simulink model "SF027A_EotProtnFwl"  (R2013b)
settings: Solver=FixedStepDiscrete  SolverMode=SingleTasking  StartTime=0.0  StopTime=1  FixedStep=0.002  RelTol=1e-3
undefined symbols (not defined in the file): ACTVREGN_CNT_U08, ARCHGLBPRM_FLOATZEROTHD_ULS_F32, EOTACTVCMDFWLREACHED_CNT_U08, EOTDMPGFWLREACHED_CNT_U08, EotProtnFwlInactvLim, EotProtnHwAgMin, EotProtnHwDegDampgX, EotProtnRackTrvlLimrRng, EotProtnSoftEndStopAuthyThd, FWLDISAD_CNT_U08, INACTVREGN_CNT_U08, MfgEnaSt1, NtcNr1, NtcSts1, sigbuilder_block
libraries: simulink x8, NxtrLim x6, FixdToFloat x5, LnrIntrpn x2, BilnrIntrpnCmnX x2, FloatToFixd x2, NxtrAbslt x1
(part 1 of 2)
Description:
  | This function sums and bounds motor torque commands from system functions whose primary input is handwheel torque.  After summation, output is limited when the signal's low-frequency content
  | exceeds calibrated boundaries.  If undesired behavior persists,  the signal-limiting strategy is replaced with implementation of a simple default assist table lookup.  Switching limiter to default table
  | occurs via Pstep/Nstep counter.  The function also outputs a scale factor for the application of additional damping.     This Function requires SF-00 Common Calibrations.
settings Model: Creator=lzz0tm  LastModifiedBy=fzx0rm
settings Model: ModifiedHistory=|
  | 001
  | Initial release
  | K. Derry
  | 18-Apr-2012
  | ICR 3358
  | 
  | 002
  | 1.  Added three limiters, applied to incoming Hysteresis_Comp, HighFreqAssist, and BaseAssistCmd.
  | 2. Created three new calibrations for input limiters.
  | 3. Increased range of boundary cals from +/- 8.8 to +/-16.
  | K. Derry
  | 31-May-2012
  | ICR 3467
  | 
  | 003
  | Extensive logic changes in model.
  | Four additional display variables.
  | K. Derry
  | 7-Jun-2012
  | ICR 3479
  | 
  | 004
  | Added logic to change AssistActiveRaw to zero when PstepNstep counter reaches saturation.
  | Changed PN Counter IF..THEN logic from “>=” to “>”.
  | K. Derry
  | 20-Jun-2012
  | ICR-3541
  | 
  | 005
  | 1. Logic now transitions output from a boundary-limited value to a default assist table lookup.
  | 2. Added new display variables.
  | 3. Increase range of boundary cals from +/-8.8 to +/-16.
  | K. Derry
  | 23-Jul-2012
  | ICR-3602
  | 
  | 006
  | Changed range & resolution of default assist cals to match Assist tables.
  | K. Derry
  | 31-Jul-2012
  | anom 3594
  | 
  | 007
  | Reduce table size and cal only quadrants 1 and 2, calculating 3 and 4.
  | Add NTC outputs to FDD to match existing code.
  | Modify model layout to better match existing code.
  | Use common vehicle speed table.
  | Eliminate Word doc.
  | K. Derry
  | 23-Jan-2013
  | ICR-3927
  | 
  | 008
  | Add inputs and logic to defeat firewall when SF-01 is using linear gain table.
  | Replace 1x12 'Cmn_t_VehSpd_Kph' with 1x8 'AsstFW_t_VehSpd_kph'.
  | Resize boundary tables to 8 vehicle speeds.
  | S. Millsap
  | K. Derry
  | 30-Apr-2013
  | ICR-4102
  | 
  | 009
  | Change rates & states execution requirement from Optional to Do Not Execute for Warm Init
  | and Disable
  | S. Millsap
  | 12-Nov-14
  | ICR-4722
settings SolverCC: AutoInsertRateTranBlk=on  InsertRTBMode=Always
settings DataIOCC: LimitDataPoints=off  SaveFormat=Structure  ReturnWorkspaceOutputs=on
settings OptimizationCC: BlockReduction=off  InlineParams=on  ZeroExternalMemoryAtStartup=off  ZeroInternalMemoryAtStartup=off  OptimizeModelRefInitCode=on  LifeSpan=1
settings DebuggingCC: SignalInfNanChecking=error  SignalRangeChecking=warning  UnderspecifiedInitializationDetection=Simplified  SolverPrmCheckMsg=error  InheritedTsInSrcMsg=error  DiscreteInheritContinuousMsg=error  SingleTaskRateTransMsg=error  TasksWithSamePriorityMsg=error  SigSpecEnsureSampleTimeMsg=error  CheckMatrixSingularityMsg=error  ParameterUnderflowMsg=error  ParameterPrecisionLossMsg=error  ParameterTunabilityLossMsg=error  FixptConstUnderflowMsg=warning  FixptConstOverflowMsg=warning  VectorMatrixConversionMsg=error  SignalLabelMismatchMsg=error  UnconnectedInputMsg=error  UnconnectedOutputMsg=error  UnconnectedLineMsg=error  SFcnCompatibilityMsg=error  UniqueDataStoreMsg=warning  BusObjectLabelMismatch=error  RootOutportRequireBusObject=error  AssertControl=DisableAll  ModelReferenceIOMsg=error  ModelReferenceVersionMismatchMessage=warning  ModelReferenceIOMismatchMessage=error  ModelReferenceCSMismatchMessage=warning  ModelReferenceDataLoggingMessage=error  StateNameClashWarn=warning  StrictBusMsg=ErrorOnBusTreatedAsVector  NonBusSignalsTreatedAsBus=error  SFUnexpectedBacktrackingDiag=error  SFInvalidInputDataAccessInChartInitDiag=error  SFNoUnconditionalDefaultTransitionDiag=error  SFTransitionOutsideNaturalParentDiag=error  SFUnconditionalTransitionShadowingDiag=error  SFUndirectedBroadcastEventsDiag=error
settings ModelReferenceCC: ModelReferenceNumInstancesAllowed=Single
settings RTWCC: SystemTargetFile=autosar.tlc  GenCodeOnly=on  TemplateMakefile=ert_default_tmf  Description=AUTOSAR  GenerateReport=on  ProcessScript=autosar_make_rtw_hook  LaunchReport=on
settings CodeAppCC: GenerateComments=off  IgnoreCustomStorageClasses=off  CustomSymbolStrType=$N$R$M  CustomSymbolStrBlkIO=$N$M  SimulinkBlockComments=off
settings STFCustomTargetCC: ParMdlRefBuildCompliant=on  CompOptLevelCompliant=on  IncludeMdlTerminateFcn=off  CombineOutputUpdateFcns=on  SuppressErrorStatus=on  ERTFirstTimeCompliant=on  ERTCustomFileBanners=on  SupportNonFinite=off  SupportComplex=off  SupportContinuousTime=off  SupportNonInlinedSFcns=off  MATLABClassNameForMDSCustomization=Simulink.SoftwareTarget.ERTCustomization  AutosarCompliant=on  GRTInterface=off  SystemTargetFile=autosar.tlc
settings ERTTargetCC: CodeReplacementLibrary=ANSI_C  ConcurrentExecutionCompliant=off  IncludeMdlTerminateFcn=off  SuppressErrorStatus=on  SupportNonFinite=off  SupportComplex=off  ModelStepFunctionPrototypeControlCompliant=off  CPPClassGenCompliant=off  AutosarCompliant=on  InlinedParameterPlacement=NonHierarchical  ERTCustomFileTemplate=example_file_process.tlc  EnableUserReplacementTypes=on

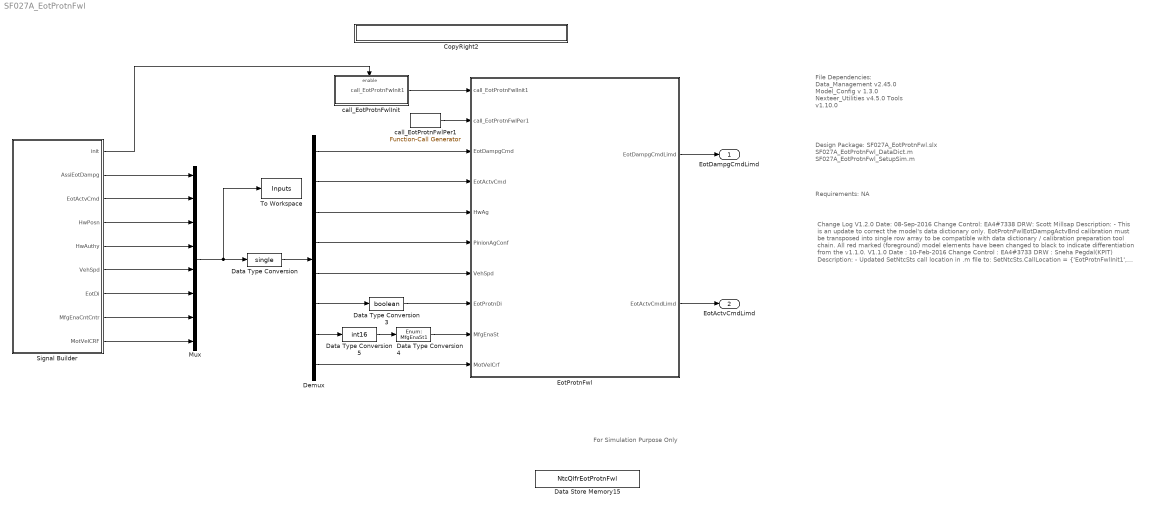
== system SF027A_EotProtnFwl ==
  note: File Dependencies:
      |
      | Data_Management v2.45.0
      | Model_Config v 1.3.0
      | Nexteer_Utilities v4.5.0
      | Tools v1.10.0
  note: Design Package:
      | SF027A_EotProtnFwl.slx
      | SF027A_EotProtnFwl_DataDict.m
      | SF027A_EotProtnFwl_SetupSim.m
  note: Change Log
      | V1.2.0
      | Date: 08-Sep-2016
      | Change Control: EA4#7338
      | DRW: Scott Millsap
      | Description:
      | - This is an update to correct the model's data dictionary only. EotProtnFwlEotDampgActvBnd
      | calibration must be transposed into single row array to be compatible with data dictionary /
      | calibration preparation tool chain.   All red marked (foreground) model elements have been changed to
      | black to indicate differentiation from the v1.1.0.
      | V1.1.0
      | Date : 10-Feb-2016
      | Change Control : EA4#3733
      | DRW : Sneha Pegdal(KPIT)
      | Description:
      | - Updated SetNtcSts call location in .m file to:
      | SetNtcSts.CallLocation = {'EotProtnFwlInit1', 'EotProtnFwlPer1'};
      | - Created an output "EotDampgFwlReached' (assigned with value 'false')
      |  from "Defeat Firewall" (If) subsystemand linked it to merge block.
      | - Renamed output "EotDampgFwlOverBnd" of "EotDmpActiveRegion"
      |   (ElseIf) subsystem to "EotDampgFwlReached'.
      | - Created an output "EotActvCmdFwlReached' (assigned with value 'false')
      |   from "Defeat Firewall1" (If) subsystem and linked it to merge block.
      | - In "Set_Faults" subsystem, removed conversion from bool to unit8. Modified logic of setting "NtcStInfo".
      |
      | Ver: 1.0.0
      | Author : KeyurKumar Gondaliya(KPIT)
      | Date : 25-Jan-2016
      | ICR- EA4#3059
      | - EA4 Initial Version from EA3 v4.0.X
  note: Requirements: NA
  note: For Simulation Purpose Only
  CopyRight2 : Subsystem  Description=|  mask(Copyright Information){none=on}
      | Copyright info block.                                               
      |                                                                     
      | Place copyright information at the top of every subsystem in design.
      mask prompts: none "No parameters"
      mask help: Place copyright information at the top of every subsystem in design.
      mask Display:
      | NxtrConf = 'Nexteer Confidential';
      | 
      | sys = bdroot; %handle for the current model ("system")
      | first = get_param(sys,'Created');
      | first = first(end-3:end);  %year is last four digits
      | 
      | last = get_param(sys,'LastModifiedDate');
      | if isempty(last)
      |     last = datestr(now,'yyyy');
      | else
      |     last = last(end-3:end);
      | end
      | 
      | if strcmp(first,last)
      |     fprintf('%s -- Copyright %s Nexteer',NxtrConf,first)
      | else
      |     fprintf('%s -- %s%s- %s Nexteer',NxtrConf,char(169),first,last)
      | end
  Data Store Memory15 : DataStoreMemory  DataStoreName=NtcQlfrEotProtnFwl  InitialValue=SigQlfr1.SIGQLFR_PASSD  OutDataTypeStr=Enum: SigQlfr1
  Data Type Conversion : DataTypeConversion  OutDataTypeStr=single
  Data Type Conversion3 : DataTypeConversion  OutDataTypeStr=boolean
  Data Type Conversion4 : DataTypeConversion  OutDataTypeStr=Enum: MfgEnaSt1
  Data Type Conversion5 : DataTypeConversion  OutDataTypeStr=int16
  Demux : Demux  Outputs=8
  EotProtnFwl : Subsystem
  Mux : Mux  Inputs=8
  Signal Builder : Subsystem  Tag=STV Subsys  LoadFcn=sigbuilder_block('load');  StartFcn=sigbuilder_block('start');  StopFcn=sigbuilder_block('stop');  ClipboardFcn=sigbuilder_block('clipboard');  mask(Sigbuilder block){}
      mask help: Simulink:masks:SigbuilderBlock_MD
      mask init:
      | if ~strcmp(get_param(bdroot(gcbh),'SimulationStatus'),'stopped') tuvar = sigbuilder_block('maskInit'); end
      settings: CopyFcn=sigbuilder_block('copy');  DeleteFcn=sigbuilder_block('delete');  ModelCloseFcn=sigbuilder_block('modelClose');  PreSaveFcn=sigbuilder_block('preSave');  PauseFcn=sigbuilder_block('pause');  ContinueFcn=sigbuilder_block('continue');  NameChangeFcn=sigbuilder_block('namechange');  OpenFcn=sigbuilder_block('open',[55.5 0 1204.5 730.5 ]);  CloseFcn=sigbuilder_block('close');
      mask Display: plot(0, 0, 100, 100,[2, 2, 32, 32, 2], [68, 8, 8, 68, 68],[32, 2], [38, 38], [32, 19, 2],[53, 60, 44], [32, 17, 17, 2],[16, 16, 31, 31]);txt = getActiveGroup(gcbh);text(2, 100, txt,'verticalAlignment', 'top');
  To Workspace : ToWorkspace  VariableName=Inputs  SampleTime=-1
  call_EotProtnFwlInit : Subsystem  TreatAsAtomicUnit=on
  call_EotProtnFwlPer1 : simulink/Ports & Subsystems/Function-Call Generator  RequirementInfo={} %GIDa_97dce53d_9879_4c16_9f7c_2c76ae6021b7  sample_time=0.002  numberOfIterations=1
  EotDampgCmdLimd : Outport
  EotActvCmdLimd : Outport  Port=2
  wires:
  call_EotProtnFwlPer1/1 -> EotProtnFwl/2(call_EotProtnFwlPer1)
  EotProtnFwl/1(EotDampgCmdLimd) -> EotDampgCmdLimd/1
  EotProtnFwl/2(EotActvCmdLimd) -> EotActvCmdLimd/1
  call_EotProtnFwlInit/1(call_EotProtnFwInit1) -> EotProtnFwl/1(call_EotProtnFwlInit1)
  Mux/1 -> To Workspace/1, Data Type Conversion/1
  Signal Builder/1(init) -> call_EotProtnFwlInit/Enable
  Signal Builder/5(HwAuthy) -> Mux/4
  Signal Builder/6(VehSpd) -> Mux/5
  Signal Builder/4(HwPosn) -> Mux/3
  Signal Builder/7(EotDi) -> Mux/6
  Signal Builder/3(EotActvCmd) -> Mux/2
  Signal Builder/8(MfgEnaCntCntr) -> Mux/7
  Signal Builder/2(AssiEotDampg) -> Mux/1
  Signal Builder/9(MotVelCRF) -> Mux/8
  Demux/1 -> EotProtnFwl/3(EotDampgCmd)
  Demux/2 -> EotProtnFwl/4(EotActvCmd)
  Demux/3 -> EotProtnFwl/5(HwAg)
  Demux/4 -> EotProtnFwl/6(PinionAgConf)
  Demux/5 -> EotProtnFwl/7(VehSpd)
  Demux/6 -> Data Type Conversion3/1
  Demux/7 -> Data Type Conversion5/1
  Demux/8 -> EotProtnFwl/10(MotVelCrf)
  Data Type Conversion/1 -> Demux/1
  Data Type Conversion3/1 -> EotProtnFwl/8(EotProtnDi)
  Data Type Conversion4/1 -> EotProtnFwl/9(MfgEnaSt)
  Data Type Conversion5/1 -> Data Type Conversion4/1

== system SF027A_EotProtnFwl/CopyRight2 ==

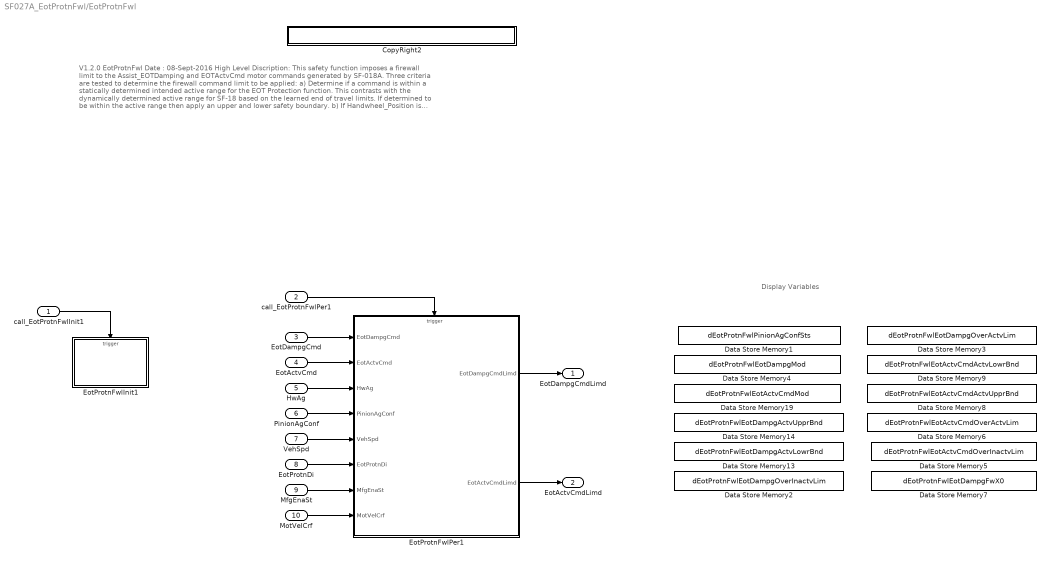
== system SF027A_EotProtnFwl/EotProtnFwl ==
  note: Display Variables
  note: V1.2.0    EotProtnFwl                                                                                                                                  Date : 08-Sept-2016
      |
      | High Level Discription:
      |
      | This safety function imposes a firewall limit to the Assist_EOTDamping and EOTActvCmd motor commands generated by SF-018A.
      |
      |  Three criteria are tested to determine the firewall command limit to be applied:
      | a) Determine if a command is within a statically determined intended active range for the EOT Protection function.  This contrasts with the
      | dynamically determined active range for SF-18 based on the learned end of travel limits. If determined to be within the active range then apply
      | an upper and lower safety boundary.
      | b) If Handwheel_Position is inboard of the active region (e.g. between +/- X0), then apply simple saturation limit.
      | c) If Handwheel_Authority is below a calibration threshold value, then apply simple saturation limit.
  call_EotProtnFwlInit1 : Inport
  call_EotProtnFwlPer1 : Inport  Port=2
  EotDampgCmd : Inport  Port=3
  EotActvCmd : Inport  Port=4
  HwAg : Inport  Port=5
  PinionAgConf : Inport  Port=6
  VehSpd : Inport  Port=7
  EotProtnDi : Inport  Port=8
  MfgEnaSt : Inport  Port=9
  MotVelCrf : Inport  Port=10
  CopyRight2 : Subsystem  Description=|  mask(Copyright Information){none=on}
      | Copyright info block.                                               
      |                                                                     
      | Place copyright information at the top of every subsystem in design.
      mask prompts: none "No parameters"
      mask help: Place copyright information at the top of every subsystem in design.
      mask Display:
      | NxtrConf = 'Nexteer Confidential';
      | 
      | sys = bdroot; %handle for the current model ("system")
      | first = get_param(sys,'Created');
      | first = first(end-3:end);  %year is last four digits
      | 
      | last = get_param(sys,'LastModifiedDate');
      | if isempty(last)
      |     last = datestr(now,'yyyy');
      | else
      |     last = last(end-3:end);
      | end
      | 
      | if strcmp(first,last)
      |     fprintf('%s -- Copyright %s Nexteer',NxtrConf,first)
      | else
      |     fprintf('%s -- %s%s- %s Nexteer',NxtrConf,char(169),first,last)
      | end
  Data Store Memory1 : DataStoreMemory  DataStoreName=dEotProtnFwlPinionAgConfSts  OutDataTypeStr=boolean  StateMustResolveToSignalObject=on
  Data Store Memory13 : DataStoreMemory  DataStoreName=dEotProtnFwlEotDampgActvLowrBnd  OutDataTypeStr=single  StateMustResolveToSignalObject=on
  Data Store Memory14 : DataStoreMemory  DataStoreName=dEotProtnFwlEotDampgActvUpprBnd  OutDataTypeStr=single  StateMustResolveToSignalObject=on
  Data Store Memory19 : DataStoreMemory  DataStoreName=dEotProtnFwlEotActvCmdMod  OutDataTypeStr=uint8  StateMustResolveToSignalObject=on
  Data Store Memory2 : DataStoreMemory  DataStoreName=dEotProtnFwlEotDampgOverInactvLim  OutDataTypeStr=boolean  StateMustResolveToSignalObject=on
  Data Store Memory3 : DataStoreMemory  DataStoreName=dEotProtnFwlEotDampgOverActvLim  OutDataTypeStr=boolean  StateMustResolveToSignalObject=on
  Data Store Memory4 : DataStoreMemory  DataStoreName=dEotProtnFwlEotDampgMod  OutDataTypeStr=uint8  StateMustResolveToSignalObject=on
  Data Store Memory5 : DataStoreMemory  DataStoreName=dEotProtnFwlEotActvCmdOverInactvLim  OutDataTypeStr=boolean  StateMustResolveToSignalObject=on
  Data Store Memory6 : DataStoreMemory  DataStoreName=dEotProtnFwlEotActvCmdOverActvLim  OutDataTypeStr=boolean  StateMustResolveToSignalObject=on
  Data Store Memory7 : DataStoreMemory  DataStoreName=dEotProtnFwlEotDampgFwX0  StateMustResolveToSignalObject=on
  Data Store Memory8 : DataStoreMemory  DataStoreName=dEotProtnFwlEotActvCmdActvUpprBnd  OutDataTypeStr=single  StateMustResolveToSignalObject=on
  Data Store Memory9 : DataStoreMemory  DataStoreName=dEotProtnFwlEotActvCmdActvLowrBnd  OutDataTypeStr=single  StateMustResolveToSignalObject=on
  EotProtnFwlInit1 : Subsystem  TreatAsAtomicUnit=on
  EotProtnFwlPer1 : Subsystem
  EotDampgCmdLimd : Outport
  EotActvCmdLimd : Outport  Port=2
  wires:
  call_EotProtnFwlInit1/1 -> EotProtnFwlInit1/Trigger
  call_EotProtnFwlPer1/1 -> EotProtnFwlPer1/Trigger
  EotProtnFwlPer1/1(EotDampgCmdLimd) -> EotDampgCmdLimd/1
  EotProtnFwlPer1/2(EotActvCmdLimd) -> EotActvCmdLimd/1
  EotDampgCmd/1 -> EotProtnFwlPer1/1(EotDampgCmd)
  EotActvCmd/1 -> EotProtnFwlPer1/2(EotActvCmd)
  HwAg/1 -> EotProtnFwlPer1/3(HwAg)
  PinionAgConf/1 -> EotProtnFwlPer1/4(PinionAgConf)
  VehSpd/1 -> EotProtnFwlPer1/5(VehSpd)
  EotProtnDi/1 -> EotProtnFwlPer1/6(EotProtnDi)
  MfgEnaSt/1 -> EotProtnFwlPer1/7(MfgEnaSt)
  MotVelCrf/1 -> EotProtnFwlPer1/8(MotVelCrf)

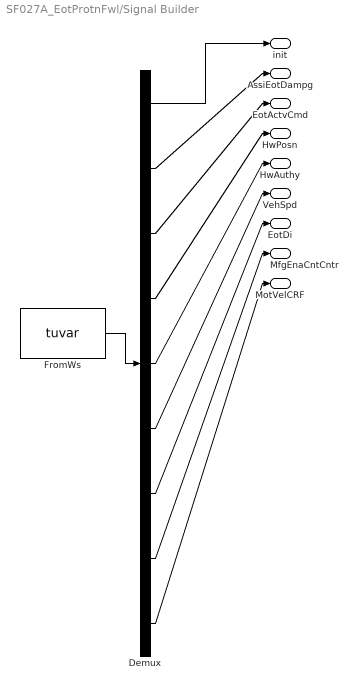
== system SF027A_EotProtnFwl/Signal Builder ==
  Demux : Demux  Tag=STV Demux  Outputs=9
  FromWs : FromWorkspace  Tag=STV FromWs  VariableName=tuvar  SampleTime=0
      SigBuilderData=|
      | common.afterFinalStr = 'Extrapolate'
      | common.sampleTime = 0
      | dataSet.timeRange = [0 5]
      | dataSet.name = 'SF027A_EotProtnFw'
      | sbobj.Name = 'Signal Builder'
      | sbobj.Groups.Name = 'SF027A_EotProtnFw'
      | sbobj.Groups.Signals(1).Name = 'init'
      | sbobj.Groups.Signals(1).XData = [0 0.002 0.004 0.006 0.008 0.01 0.012 0.014 0.016 0.018 0.02 0.022 ... (2501 elements, 1x2501)]
      | sbobj.Groups.Signals(1).YData = [1 0 0 0 0 0 0 0 0 0 0 0 ... (2501 elements, 1x2501)]
      | sbobj.Groups.Signals(2).Name = 'AssiEotDampg'
      | sbobj.Groups.Signals(2).XData = [0 0.002 0.004 0.006 0.008 0.01 0.012 0.014 0.016 0.018 0.02 0.022 ... (2501 elements, 1x2501)]
      | sbobj.Groups.Signals(2).YData = [0 0.0175999882667 0.0351999061334 0.0527996832006 0.0703992490691 0.0879985333407 0.105597465618 0.123195975506 0.14079399261 0.158391446539 0.175988266901 0.193584383311 ... (2501 elements, 1x2501)]
      | sbobj.Groups.Signals(3).Name = 'EotActvCmd'
      | sbobj.Groups.Signals(3).XData = [0 0.002 0.004 0.006 0.008 0.01 0.012 0.014 0.016 0.018 0.02 0.022 ... (2501 elements, 1x2501)]
      | sbobj.Groups.Signals(3).YData = [0 0.0175999882667 0.0351999061334 0.0527996832006 0.0703992490691 0.0879985333407 0.105597465618 0.123195975506 0.14079399261 0.158391446539 0.175988266901 0.193584383311 ... (2501 elements, 1x2501)]
      | sbobj.Groups.Signals(4).Name = 'HwPosn'
      | sbobj.Groups.Signals(4).XData = [0 0.002 0.004 0.006 0.008 0.01 0.012 0.014 0.016 0.018 0.02 0.022 ... (2501 elements, 1x2501)]
      | sbobj.Groups.Signals(4).YData = [0 2.87999808 5.75998464001 8.63994816009 11.5198771204 14.3997600012 17.279585283 20.1593414465 23.0390169726 25.9186003427 28.7980800384 31.6774445418 ... (2501 elements, 1x2501)]
      | sbobj.Groups.Signals(5).Name = 'HwAuthy'
      | sbobj.Groups.Signals(5).XData = [0 0.002 0.004 0.006 0.008 0.01 0.012 0.014 0.016 0.018 0.02 0.022 ... (2501 elements, 1x2501)]
      | sbobj.Groups.Signals(5).YData = [0 1 0 1 0 1 0 1 0 1 0 1 ... (2501 elements, 1x2501)]
      | sbobj.Groups.Signals(6).Name = 'VehSpd'
      | sbobj.Groups.Signals(6).XData = [0 0.002 0.004 0.006 0.008 0.01 0.012 0.014 0.016 0.018 0.02 0.022 ... (2501 elements, 1x2501)]
      | sbobj.Groups.Signals(6).YData = [1.02199931867 2.04399454934 3.06598160403 4.08795639481 5.10991483376 6.13185283306 7.15376630496 8.1756511618 9.19750331605 10.2193186803 11.2410931673 12.2628226899 ... (2501 elements, 1x2501)]
      | sbobj.Groups.Signals(7).Name = 'EotDi'
      | sbobj.Groups.Signals(7).XData = [0 0.002 0.004 0.006 0.008 0.01 0.012 0.014 0.016 0.018 0.02 0.022 ... (2501 elements, 1x2501)]
      | sbobj.Groups.Signals(7).YData = [0 1 0 1 0 1 0 1 0 1 0 1 ... (2501 elements, 1x2501)]
      | sbobj.Groups.Signals(8).Name = 'MfgEnaCntCntr'
      | sbobj.Groups.Signals(8).XData = [0 2 2 3 3 5]
      | sbobj.Groups.Signals(8).YData = [0 0 1 1 0 0]
      | sbobj.Groups.Signals(9).Name = 'MotVelCRF'
      | sbobj.Groups.Signals(9).XData = [0 0.002 0.004 0.006 0.008 0.01 0.012 0.014 0.016 0.018 0.02 0.022 ... (2501 elements, 1x2501)]
      | sbobj.Groups.Signals(9).YData = [2.23599850933 4.47198807468 6.70795975207 8.94390459764 11.1798136676 13.4156780183 15.6514887063 17.8872367884 20.1229133216 22.3585093631 24.5940159707 26.8294242022 ... (2501 elements, 1x2501)]
      | sbobj.Groups.TimeRange = [0 5]
  init : Outport
  AssiEotDampg : Outport  Tag=STV Outport  Port=2
  EotActvCmd : Outport  Tag=STV Outport  Port=3
  HwPosn : Outport  Tag=STV Outport  Port=4
  HwAuthy : Outport  Tag=STV Outport  Port=5
  VehSpd : Outport  Tag=STV Outport  Port=6
  EotDi : Outport  Tag=STV Outport  Port=7
  MfgEnaCntCntr : Outport  Tag=STV Outport  Port=8
  MotVelCRF : Outport  Tag=STV Outport  Port=9
  wires:
  Demux/1 -> init/1
  FromWs/1 -> Demux/1
  Demux/2 -> AssiEotDampg/1
  Demux/3 -> EotActvCmd/1
  Demux/4 -> HwPosn/1
  Demux/5 -> HwAuthy/1
  Demux/6 -> VehSpd/1
  Demux/7 -> EotDi/1
  Demux/8 -> MfgEnaCntCntr/1
  Demux/9 -> MotVelCRF/1

== system SF027A_EotProtnFwl/call_EotProtnFwlInit ==
  Enable : EnablePort
  CopyRight2 : Subsystem  Description=|  mask(Copyright Information){none=on}
      | Copyright info block.                                               
      |                                                                     
      | Place copyright information at the top of every subsystem in design.
      mask prompts: none "No parameters"
      mask help: Place copyright information at the top of every subsystem in design.
      mask Display:
      | NxtrConf = 'Nexteer Confidential';
      | 
      | sys = bdroot; %handle for the current model ("system")
      | first = get_param(sys,'Created');
      | first = first(end-3:end);  %year is last four digits
      | 
      | last = get_param(sys,'LastModifiedDate');
      | if isempty(last)
      |     last = datestr(now,'yyyy');
      | else
      |     last = last(end-3:end);
      | end
      | 
      | if strcmp(first,last)
      |     fprintf('%s -- Copyright %s Nexteer',NxtrConf,first)
      | else
      |     fprintf('%s -- %s%s- %s Nexteer',NxtrConf,char(169),first,last)
      | end
  call_EotProtnFwInit : simulink/Ports & Subsystems/Function-Call Generator  sample_time=0  numberOfIterations=1
  call_EotProtnFwInit1 : Outport
  wires:
  call_EotProtnFwInit/1 -> call_EotProtnFwInit1/1

== system SF027A_EotProtnFwl/EotProtnFwl/CopyRight2 ==

== system SF027A_EotProtnFwl/EotProtnFwl/EotProtnFwlInit1 ==
  note: NEXTEER TROUBLE CODES
      |
      | Number                TYPE                   Name
      | NTCNR_0X0C6      F3      NTCNumber.NTC_EotProtnFwlFlt
  function : TriggerPort  TriggerType=function-call
  Constant7 : Constant  RequirementInfo={} %GIDa_126a797a_30b9_4b52_8911_b7affaa2f3a8  Value=0  OutDataTypeStr=uint8
  CopyRight2 : Subsystem  Description=|  mask(Copyright Information){none=on}
      | Copyright info block.                                               
      |                                                                     
      | Place copyright information at the top of every subsystem in design.
      mask prompts: none "No parameters"
      mask help: Place copyright information at the top of every subsystem in design.
      mask Display:
      | NxtrConf = 'Nexteer Confidential';
      | 
      | sys = bdroot; %handle for the current model ("system")
      | first = get_param(sys,'Created');
      | first = first(end-3:end);  %year is last four digits
      | 
      | last = get_param(sys,'LastModifiedDate');
      | if isempty(last)
      |     last = datestr(now,'yyyy');
      | else
      |     last = last(end-3:end);
      | end
      | 
      | if strcmp(first,last)
      |     fprintf('%s -- Copyright %s Nexteer',NxtrConf,first)
      | else
      |     fprintf('%s -- %s%s- %s Nexteer',NxtrConf,char(169),first,last)
      | end
  Enumerated Constant4 : simulink/Sources/Enumerated Constant  RequirementInfo={} %GIDa_605febc4_2a20_461f_8109_182131f61dc1  OutDataTypeStr=Enum: NtcSts1  Value=NtcSts1.NTCSTS_PASSD  SampleTime=inf
  EotProtnFwlFlt : simulink/Sources/Enumerated Constant  RequirementInfo={} %GIDa_6290572b_f437_4fd8_9e79_bb4e9500ca68  OutDataTypeStr=Enum: NtcNr1  Value=NtcNr1.NTCNR_0X0C6  SampleTime=inf
  Ground : Ground
  SetNtcSts : Subsystem  mask(SetNTC){}
      mask help: SetNTC library block
  wires:
  EotProtnFwlFlt/1 -> SetNtcSts/1(NtcNr)
  Constant7/1 -> SetNtcSts/2(NtcStInfo)
  Enumerated Constant4/1 -> SetNtcSts/3(NtcSts)
  Ground/1 -> SetNtcSts/4(DebStep)

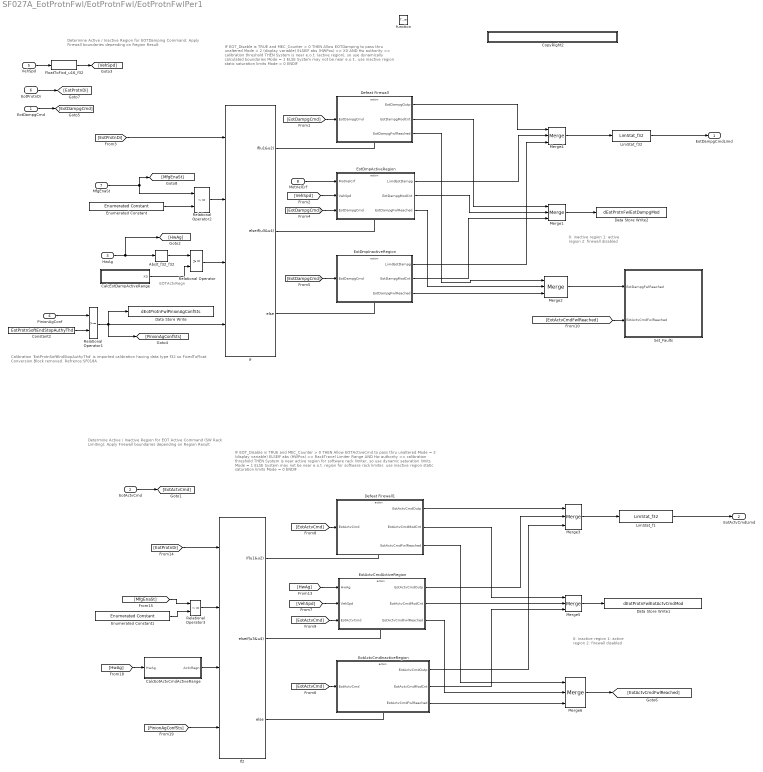
== system SF027A_EotProtnFwl/EotProtnFwl/EotProtnFwlPer1 ==
  note: Calibration 'EotProtnSoftEndStopAuthyThd' is imported calibration having data type f32 so FixedToFloat
      | Conversion Block removed.
      |
      | Refrence:SF018A
  note: EOTActvRegn
  note: 0: inactive region
      | 1: active region
      | 2: firewall disabled
  note: IF EOT_Disable is TRUE and MEC_Counter > 0 THEN
      |      Allow EOTDamping  to pass thru unaltered
      |      Mode = 2 (display variable)
      | ELSEIF abs (HWPos) >= X0   AND   Hw authority >= calibration threshold THEN
      |      System is near e.o.t. (active region), so use dynamically calculated boundaries
      |      Mode = 1
      | ELSE
      |      System may not be near e.o.t., use inactive region static saturation limits
      |      Mode = 0
      | ENDIF
  note: IF EOT_Disable is TRUE and MEC_Counter > 0 THEN
      |      Allow EOTActiveCmd  to pass thru unaltered
      |      Mode = 2 (display variable)
      | ELSEIF abs (HWPos) >= RackTravel Limiter Range   AND  Hw authority >= calibration threshold THEN
      |      System is near active region for software rack limiter, so use dynamic saturation limits
      |      Mode = 1
      | ELSE
      |      System may not be near e.o.t. region for software rack limiter, use inactive region static saturation limits
      |      Mode = 0
      | ENDIF
  note: Determine Active / Inactive Region for
      | EOTDamping Command; Apply Firewall boundaries
      | depending on Region Result
  note: Determine Active / Inactive Region for
      | EOT Active Command (SW Rack Limiting);
      | Apply Firewall boundaries depending on Region Result
  note: 0: inactive region
      | 1: active region
      | 2: firewall disabled
  EotDampgCmd : Inport
  EotActvCmd : Inport  Port=2
  HwAg : Inport  Port=3
  PinionAgConf : Inport  Port=4
  VehSpd : Inport  Port=5
  EotProtnDi : Inport  Port=6
  MfgEnaSt : Inport  Port=7
  MotVelCrf : Inport  Port=8
  function : TriggerPort  TriggerType=function-call
  Abslt_f32_f32 : NxtrAbslt/Abslt_f32_f32  SFunctionSpec=single y1 = Abslt_f32_f32(single u1)
      settings: AttributesFormatString=%<Name>
  CalcEotActvCmdActiveRange : Subsystem
  CalcEotDampActiveRange : Subsystem
  Constant2 : Constant  Value=EotProtnSoftEndStopAuthyThd
  CopyRight2 : Subsystem  Description=|  mask(Copyright Information){none=on}
      | Copyright info block.                                               
      |                                                                     
      | Place copyright information at the top of every subsystem in design.
      mask prompts: none "No parameters"
      mask help: Place copyright information at the top of every subsystem in design.
      mask Display:
      | NxtrConf = 'Nexteer Confidential';
      | 
      | sys = bdroot; %handle for the current model ("system")
      | first = get_param(sys,'Created');
      | first = first(end-3:end);  %year is last four digits
      | 
      | last = get_param(sys,'LastModifiedDate');
      | if isempty(last)
      |     last = datestr(now,'yyyy');
      | else
      |     last = last(end-3:end);
      | end
      | 
      | if strcmp(first,last)
      |     fprintf('%s -- Copyright %s Nexteer',NxtrConf,first)
      | else
      |     fprintf('%s -- %s%s- %s Nexteer',NxtrConf,char(169),first,last)
      | end
  Data Store Write : DataStoreWrite  DataStoreName=dEotProtnFwlPinionAgConfSts
  Data Store Write1 : DataStoreWrite  DataStoreName=dEotProtnFwlEotActvCmdMod
  Data Store Write2 : DataStoreWrite  DataStoreName=dEotProtnFwlEotDampgMod
  Defeat Firewall : Subsystem  TreatAsAtomicUnit=on
  Defeat Firewall1 : Subsystem  TreatAsAtomicUnit=on
  Enumerated Constant : simulink/Sources/Enumerated Constant  OutDataTypeStr=Enum: MfgEnaSt1  Value=MfgEnaSt1.MFGENAST_PRDNMOD  SampleTime=inf
  Enumerated Constant1 : simulink/Sources/Enumerated Constant  OutDataTypeStr=Enum: MfgEnaSt1  Value=MfgEnaSt1.MFGENAST_PRDNMOD  SampleTime=inf
  EotActvCmdActiveRegion : Subsystem  TreatAsAtomicUnit=on
  EotActvCmdInactiveRegion : Subsystem  TreatAsAtomicUnit=on
  EotDmpActiveRegion : Subsystem  TreatAsAtomicUnit=on
  EotDmpInactiveRegion : Subsystem  TreatAsAtomicUnit=on
  FloatToFixd_u16_f32 : FloatToFixd/FloatToFixd_u16_f32  Param1=7
  If : If  NumInputs=4  IfExpression=u1&u2  ElseIfExpressions=u3&u4
  If2 : If  NumInputs=4  IfExpression=u1&u2  ElseIfExpressions=u3&u4
  LimStat_f1 : NxtrLim/LimStat_f32  LoLim=SYSGLBPRM_MOTTQCMDLOLIM_MOTNWTMTR_F32  HiLim=SYSGLBPRM_MOTTQCMDHILIM_MOTNWTMTR_F32
      settings: AttributesFormatString=|
      | Low Limit: %<LoLim>
      | High Limit:%<HiLim>
  LimStat_f32 : NxtrLim/LimStat_f32  LoLim=SYSGLBPRM_MOTTQCMDLOLIM_MOTNWTMTR_F32  HiLim=SYSGLBPRM_MOTTQCMDHILIM_MOTNWTMTR_F32
      settings: AttributesFormatString=|
      | Low Limit: %<LoLim>
      | High Limit:%<HiLim>
  Merge{1..6} (6 alike) : Merge  Inputs=3
  Relational Operator : RelationalOperator  OutDataTypeStr=boolean
  Relational Operator1 : RelationalOperator  OutDataTypeStr=boolean
  Relational Operator2 : RelationalOperator  Operator=~=  OutDataTypeStr=boolean
  Relational Operator3 : RelationalOperator  Operator=~=  OutDataTypeStr=boolean
  Set_Faults : Subsystem
  EotDampgCmdLimd : Outport
  EotActvCmdLimd : Outport  Port=2
  wires:
  If/2 -> EotDmpActiveRegion/Action
  Merge2/1 -> Set_Faults/1(EotDampgFwlReached)
  [EotActvCmdFwlReached] -> Set_Faults/2(EotActvCmdFwlReached)
  Abslt_f32_f32/1 -> Relational Operator/1
  If/3 -> EotDmpInactiveRegion/Action
  LimStat_f1/1 -> EotActvCmdLimd/1
  MotVelCrf/1 -> EotDmpActiveRegion/1(MotVelCrf)
  [VehSpd] -> EotDmpActiveRegion/2(VehSpd)
  [EotDampgCmd] -> EotDmpActiveRegion/3(EotDampgCmd)
  [EotActvCmd] -> Defeat Firewall1/1(EotActvCmd)
  [EotActvCmd] -> EotActvCmdActiveRegion/3(EotActvCmd)
  [EotDampgCmd] -> EotDmpInactiveRegion/1(EotDampgCmd)
  CalcEotDampActiveRange/1(X0) -> Relational Operator/2
  Merge1/1 -> Data Store Write2/1
  If2/2 -> EotActvCmdActiveRegion/Action
  If2/3 -> EotActvCmdInactiveRegion/Action
  [HwAg] -> EotActvCmdActiveRegion/1(HwAg)
  [VehSpd] -> EotActvCmdActiveRegion/2(VehSpd)
  Merge5/1 -> Data Store Write1/1
  [PinionAgConfSts] -> If2/4
  Merge3/1 -> LimStat_f1/1
  [HwAg] -> CalcEotActvCmdActiveRange/1(HwAg)
  CalcEotActvCmdActiveRange/1("ActvRegn ") -> If2/3
  Enumerated Constant1/1 -> Relational Operator3/2
  If/1 -> Defeat Firewall/Action
  Relational Operator2/1 -> If/2
  [EotProtnDi] -> If/1
  Relational Operator/1 -> If/3
  Relational Operator1/1 -> [PinionAgConfSts], Data Store Write/1, If/4
  [EotProtnDi] -> If2/1
  Relational Operator3/1 -> If2/2
  [EotDampgCmd] -> Defeat Firewall/1(EotDampgCmd)
  If2/1 -> Defeat Firewall1/Action
  Enumerated Constant/1 -> Relational Operator2/2
  HwAg/1 -> [HwAg], Abslt_f32_f32/1
  PinionAgConf/1 -> Relational Operator1/1
  Constant2/1 -> Relational Operator1/2
  MfgEnaSt/1 -> Relational Operator2/1, [MfgEnaSt]
  [MfgEnaSt] -> Relational Operator3/1
  VehSpd/1 -> FloatToFixd_u16_f32/1
  FloatToFixd_u16_f32/1 -> [VehSpd]
  EotProtnDi/1 -> [EotProtnDi]
  EotDampgCmd/1 -> [EotDampgCmd]
  LimStat_f32/1 -> EotDampgCmdLimd/1
  Merge4/1 -> LimStat_f32/1
  Defeat Firewall/1(EotDampgOutp) -> Merge4/1
  EotDmpActiveRegion/1(LimdEotDampg) -> Merge4/2
  EotDmpInactiveRegion/1(LimdEotDampg) -> Merge4/3
  Defeat Firewall/2(EotDampgModCnt) -> Merge1/1
  EotDmpActiveRegion/2(EotDampgModCnt) -> Merge1/2
  EotDmpInactiveRegion/2(EotDampgModCnt) -> Merge1/3
  EotActvCmd/1 -> [EotActvCmd]
  [EotActvCmd] -> EotActvCmdInactiveRegion/1(EotActvCmd)
  Defeat Firewall1/1(EotActvCmdOutp) -> Merge3/1
  EotActvCmdActiveRegion/1(EotActvCmdOutp) -> Merge3/2
  EotActvCmdInactiveRegion/1(EotActvCmdOutp) -> Merge3/3
  Defeat Firewall1/2(EotActvCmdModCnt) -> Merge5/1
  EotActvCmdActiveRegion/2(EotActvCmdModCnt) -> Merge5/2
  EotActvCmdInactiveRegion/2(EotActvCmdModCnt) -> Merge5/3
  Merge6/1 -> [EotActvCmdFwlReached]
  Defeat Firewall/3(EotDampgFwlReached) -> Merge2/1
  EotDmpActiveRegion/3(EotDampgFwlReached) -> Merge2/2
  EotDmpInactiveRegion/3(EotDampgFwlReached) -> Merge2/3
  Defeat Firewall1/3(EotActvCmdFwlReached) -> Merge6/1
  EotActvCmdActiveRegion/3(EotActvCmdFwlReached) -> Merge6/2
  EotActvCmdInactiveRegion/3(EotActvCmdFwlReached) -> Merge6/3

== system SF027A_EotProtnFwl/call_EotProtnFwlInit/CopyRight2 ==

== system SF027A_EotProtnFwl/EotProtnFwl/EotProtnFwlInit1/CopyRight2 ==

== system SF027A_EotProtnFwl/EotProtnFwl/EotProtnFwlInit1/SetNtcSts ==
  NtcNr : Inport
  NtcStInfo : Inport  Port=2
  NtcSts : Inport  Port=3
  DebStep : Inport  Port=4
  SetNtcSts : Subsystem  RequirementInfo={} %GIDa_468e1686_8a6c_4215_af7a_5797695cdce1  TreatAsAtomicUnit=on
      settings: RTWSystemCode=Inline
  wires:
  NtcNr/1 -> SetNtcSts/1(NtcNr)  "NtcNr"
  NtcSts/1 -> SetNtcSts/3(NtcSts)
  DebStep/1 -> SetNtcSts/4(DebStep)
  NtcStInfo/1 -> SetNtcSts/2(NtcStInfo)

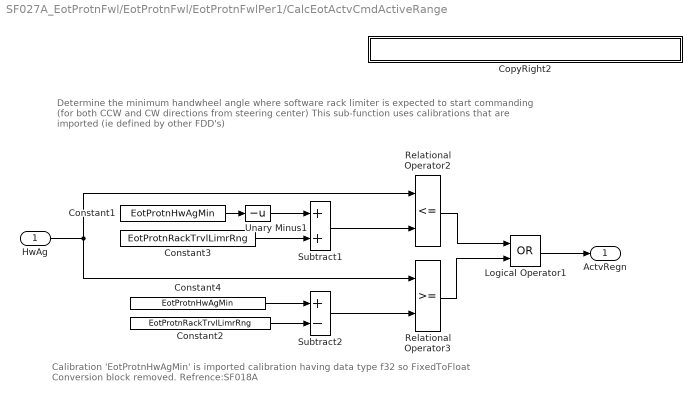
== system SF027A_EotProtnFwl/EotProtnFwl/EotProtnFwlPer1/CalcEotActvCmdActiveRange ==
  note: Determine the minimum handwheel angle where software rack limiter is expected to start commanding
      | (for both CCW and CW directions from steering center)
      |
      | This sub-function uses calibrations that are imported (ie defined by other FDD's)
  note: Calibration 'EotProtnHwAgMin' is imported calibration having data type f32 so FixedToFloat
      | Conversion block removed.
      |
      | Refrence:SF018A
  HwAg : Inport
  Constant1 : Constant  Value=EotProtnHwAgMin
  Constant2 : Constant  Value=EotProtnRackTrvlLimrRng
  Constant3 : Constant  Value=EotProtnRackTrvlLimrRng
  Constant4 : Constant  Value=EotProtnHwAgMin
  CopyRight2 : Subsystem  Description=|  mask(Copyright Information){none=on}
      | Copyright info block.                                               
      |                                                                     
      | Place copyright information at the top of every subsystem in design.
      mask prompts: none "No parameters"
      mask help: Place copyright information at the top of every subsystem in design.
      mask Display:
      | NxtrConf = 'Nexteer Confidential';
      | 
      | sys = bdroot; %handle for the current model ("system")
      | first = get_param(sys,'Created');
      | first = first(end-3:end);  %year is last four digits
      | 
      | last = get_param(sys,'LastModifiedDate');
      | if isempty(last)
      |     last = datestr(now,'yyyy');
      | else
      |     last = last(end-3:end);
      | end
      | 
      | if strcmp(first,last)
      |     fprintf('%s -- Copyright %s Nexteer',NxtrConf,first)
      | else
      |     fprintf('%s -- %s%s- %s Nexteer',NxtrConf,char(169),first,last)
      | end
  Logical Operator1 : Logic  Operator=OR  AllPortsSameDT=off  OutDataTypeStr=boolean
  Relational Operator2 : RelationalOperator  Operator=<=  OutDataTypeStr=boolean
  Relational Operator3 : RelationalOperator  OutDataTypeStr=boolean
  Subtract1 : Sum
  Subtract2 : Sum  Inputs=+-
  Unary Minus1 : UnaryMinus
  "ActvRegn " : Outport
  wires:
  Relational Operator3/1 -> Logical Operator1/2
  HwAg/1 -> Relational Operator2/1, Relational Operator3/1
  Relational Operator2/1 -> Logical Operator1/1
  Subtract1/1 -> Relational Operator2/2
  Constant3/1 -> Subtract1/2
  Constant2/1 -> Subtract2/2
  Subtract2/1 -> Relational Operator3/2
  Logical Operator1/1 -> "ActvRegn "/1
  Constant1/1 -> Unary Minus1/1
  Constant4/1 -> Subtract2/1
  Unary Minus1/1 -> Subtract1/1

== system SF027A_EotProtnFwl/EotProtnFwl/EotProtnFwlPer1/CalcEotDampActiveRange ==
  note: The innermost (closest to steering angle center) calibration point for the start of the EOT active range is computed by indexing into the
      | calibration table t2_EOTPosDepDmpXTbl for the X0 point.  This calibration is then subtracted from the k_MinRackTrvl calibration
      |
      | This sub-function uses calibrations that are imported (ie defined by other FDD's)
  note: Note: for software implementation this calibration needs to use the
      |  0 index (pull out the X0 point) from the lookup table EotProtnHwDegDampgX.
  Add : Sum  Inputs=+-
  Constant1 : Constant  Value=EotProtnHwAgMin
  Constant2 : Constant  Value=EotProtnHwDegDampgX  VectorParams1D=off
  CopyRight2 : Subsystem  Description=|  mask(Copyright Information){none=on}
      | Copyright info block.                                               
      |                                                                     
      | Place copyright information at the top of every subsystem in design.
      mask prompts: none "No parameters"
      mask help: Place copyright information at the top of every subsystem in design.
      mask Display:
      | NxtrConf = 'Nexteer Confidential';
      | 
      | sys = bdroot; %handle for the current model ("system")
      | first = get_param(sys,'Created');
      | first = first(end-3:end);  %year is last four digits
      | 
      | last = get_param(sys,'LastModifiedDate');
      | if isempty(last)
      |     last = datestr(now,'yyyy');
      | else
      |     last = last(end-3:end);
      | end
      | 
      | if strcmp(first,last)
      |     fprintf('%s -- Copyright %s Nexteer',NxtrConf,first)
      | else
      |     fprintf('%s -- %s%s- %s Nexteer',NxtrConf,char(169),first,last)
      | end
  Data Store Write : DataStoreWrite  DataStoreName=dEotProtnFwlEotDampgFwX0
  FixdToFloat_f32_u1 : FixdToFloat/FixdToFloat_f32_u16  Param1=4
  Selector : Selector  NumberOfDimensions=2  IndexMode=Zero-based  InputPortWidth=3  IndexOptions=Index vector (dialog),Index vector (dialog)  Indices=[0],0  OutputSizes=1,1
  X0 : Outport
  wires:
  Constant1/1 -> Add/1
  Add/1 -> X0/1, Data Store Write/1
  Constant2/1 -> Selector/1
  Selector/1 -> FixdToFloat_f32_u1/1
  FixdToFloat_f32_u1/1 -> Add/2

== system SF027A_EotProtnFwl/EotProtnFwl/EotProtnFwlPer1/CopyRight2 ==

== system SF027A_EotProtnFwl/EotProtnFwl/EotProtnFwlPer1/Defeat Firewall ==
  EotDampgCmd : Inport
  Action Port : ActionPort  ActionType=then
  Constant1 : Constant  Value=false  OutDataTypeStr=boolean
      settings: AttributesFormatString=%<OutDataTypeStr>
  Constant8 : Constant  Value=FWLDISAD_CNT_U08  OutDataTypeStr=uint8
      settings: AttributesFormatString=%<OutDataTypeStr>
  CopyRight2 : Subsystem  Description=|  mask(Copyright Information){none=on}
      | Copyright info block.                                               
      |                                                                     
      | Place copyright information at the top of every subsystem in design.
      mask prompts: none "No parameters"
      mask help: Place copyright information at the top of every subsystem in design.
      mask Display:
      | NxtrConf = 'Nexteer Confidential';
      | 
      | sys = bdroot; %handle for the current model ("system")
      | first = get_param(sys,'Created');
      | first = first(end-3:end);  %year is last four digits
      | 
      | last = get_param(sys,'LastModifiedDate');
      | if isempty(last)
      |     last = datestr(now,'yyyy');
      | else
      |     last = last(end-3:end);
      | end
      | 
      | if strcmp(first,last)
      |     fprintf('%s -- Copyright %s Nexteer',NxtrConf,first)
      | else
      |     fprintf('%s -- %s%s- %s Nexteer',NxtrConf,char(169),first,last)
      | end
  EotDampgOutp : Outport
  EotDampgModCnt : Outport  Port=2
  EotDampgFwlReached : Outport  Port=3
  wires:
  Constant8/1 -> EotDampgModCnt/1
  EotDampgCmd/1 -> EotDampgOutp/1
  Constant1/1 -> EotDampgFwlReached/1

== system SF027A_EotProtnFwl/EotProtnFwl/EotProtnFwlPer1/Defeat Firewall1 ==
  EotActvCmd : Inport
  Action Port : ActionPort  ActionType=then
  Constant1 : Constant  Value=false  OutDataTypeStr=boolean
      settings: AttributesFormatString=%<OutDataTypeStr>
  Constant6 : Constant  Value=FWLDISAD_CNT_U08  OutDataTypeStr=uint8
      settings: AttributesFormatString=%<OutDataTypeStr>
  CopyRight2 : Subsystem  Description=|  mask(Copyright Information){none=on}
      | Copyright info block.                                               
      |                                                                     
      | Place copyright information at the top of every subsystem in design.
      mask prompts: none "No parameters"
      mask help: Place copyright information at the top of every subsystem in design.
      mask Display:
      | NxtrConf = 'Nexteer Confidential';
      | 
      | sys = bdroot; %handle for the current model ("system")
      | first = get_param(sys,'Created');
      | first = first(end-3:end);  %year is last four digits
      | 
      | last = get_param(sys,'LastModifiedDate');
      | if isempty(last)
      |     last = datestr(now,'yyyy');
      | else
      |     last = last(end-3:end);
      | end
      | 
      | if strcmp(first,last)
      |     fprintf('%s -- Copyright %s Nexteer',NxtrConf,first)
      | else
      |     fprintf('%s -- %s%s- %s Nexteer',NxtrConf,char(169),first,last)
      | end
  EotActvCmdOutp : Outport
  EotActvCmdModCnt : Outport  Port=2
  EotActvCmdFwlReached : Outport  Port=3
  wires:
  Constant6/1 -> EotActvCmdModCnt/1
  EotActvCmd/1 -> EotActvCmdOutp/1
  Constant1/1 -> EotActvCmdFwlReached/1

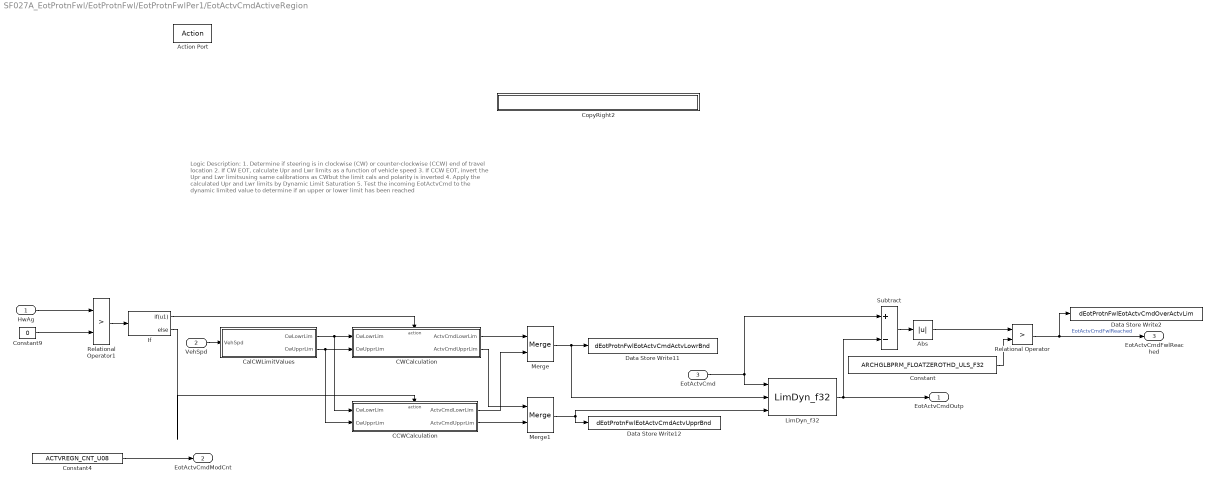
== system SF027A_EotProtnFwl/EotProtnFwl/EotProtnFwlPer1/EotActvCmdActiveRegion ==
  note: Logic Description:
      | 1. Determine if steering is in clockwise (CW) or counter-clockwise (CCW) end of travel location
      | 2. If CW EOT, calculate Upr and Lwr limits as a function of vehicle speed
      | 3. If CCW EOT, invert the Upr and Lwr limitsusing same calibrations as CWbut the limit cals and polarity is inverted
      | 4. Apply the calculated Upr and Lwr limits by Dynamic Limit Saturation
      | 5. Test the incoming EotActvCmd to the dynamic limited value to determine if an upper or lower limit has been reached
  HwAg : Inport
  VehSpd : Inport  Port=2
  EotActvCmd : Inport  Port=3
  Action Port : ActionPort  ActionType=elseif
  Abs : Abs
  CCWCalculation : Subsystem  TreatAsAtomicUnit=on
  CWCalculation : Subsystem  TreatAsAtomicUnit=on
  CalCWLimitValues : Subsystem
  Constant : Constant  Value=ARCHGLBPRM_FLOATZEROTHD_ULS_F32
  Constant4 : Constant  Value=ACTVREGN_CNT_U08  OutDataTypeStr=uint8
      settings: AttributesFormatString=%<OutDataTypeStr>
  Constant9 : Constant  Value=0  VectorParams1D=off
  CopyRight2 : Subsystem  Description=|  mask(Copyright Information){none=on}
      | Copyright info block.                                               
      |                                                                     
      | Place copyright information at the top of every subsystem in design.
      mask prompts: none "No parameters"
      mask help: Place copyright information at the top of every subsystem in design.
      mask Display:
      | NxtrConf = 'Nexteer Confidential';
      | 
      | sys = bdroot; %handle for the current model ("system")
      | first = get_param(sys,'Created');
      | first = first(end-3:end);  %year is last four digits
      | 
      | last = get_param(sys,'LastModifiedDate');
      | if isempty(last)
      |     last = datestr(now,'yyyy');
      | else
      |     last = last(end-3:end);
      | end
      | 
      | if strcmp(first,last)
      |     fprintf('%s -- Copyright %s Nexteer',NxtrConf,first)
      | else
      |     fprintf('%s -- %s%s- %s Nexteer',NxtrConf,char(169),first,last)
      | end
  Data Store Write11 : DataStoreWrite  DataStoreName=dEotProtnFwlEotActvCmdActvLowrBnd
  Data Store Write12 : DataStoreWrite  DataStoreName=dEotProtnFwlEotActvCmdActvUpprBnd
  Data Store Write2 : DataStoreWrite  DataStoreName=dEotProtnFwlEotActvCmdOverActvLim
  If : If  IfExpression=u1
  LimDyn_f32 : NxtrLim/LimDyn_f32
  Merge : Merge
  Merge1 : Merge
  Relational Operator : RelationalOperator  Operator=>  OutDataTypeStr=boolean
  Relational Operator1 : RelationalOperator  Operator=>  OutDataTypeStr=boolean
  Subtract : Sum  Inputs=+-
  EotActvCmdOutp : Outport
  EotActvCmdModCnt : Outport  Port=2  InitialOutput=1
  EotActvCmdFwlReached : Outport  Port=3
      settings: AttributesFormatString=%<Tag>
  wires:
  HwAg/1 -> Relational Operator1/1
  Relational Operator/1 -> Data Store Write2/1, EotActvCmdFwlReached/1  "EotActvCmdFwlReached"
  Constant4/1 -> EotActvCmdModCnt/1
  Constant9/1 -> Relational Operator1/2
  Relational Operator1/1 -> If/1
  EotActvCmd/1 -> Subtract/1, LimDyn_f32/1
  Merge/1 -> LimDyn_f32/2, Data Store Write11/1
  Merge1/1 -> LimDyn_f32/3, Data Store Write12/1
  LimDyn_f32/1 -> Subtract/2, EotActvCmdOutp/1
  VehSpd/1 -> CalCWLimitValues/1(VehSpd)
  Subtract/1 -> Abs/1
  Abs/1 -> Relational Operator/1
  Constant/1 -> Relational Operator/2
  If/1 -> CWCalculation/Action
  If/2 -> CCWCalculation/Action
  CWCalculation/1(ActvCmdLowrLim) -> Merge/1
  CCWCalculation/1(ActvCmdLowrLim) -> Merge/2
  CWCalculation/2(ActvCmdUpprLim) -> Merge1/1
  CCWCalculation/2(ActvCmdUpprLim) -> Merge1/2
  CalCWLimitValues/1(CwLowrLim) -> CWCalculation/1(CwLowrLim), CCWCalculation/1(CwLowrLim)
  CalCWLimitValues/2(CwUpprLim) -> CWCalculation/2(CwUpprLim), CCWCalculation/2(CwUpprLim)

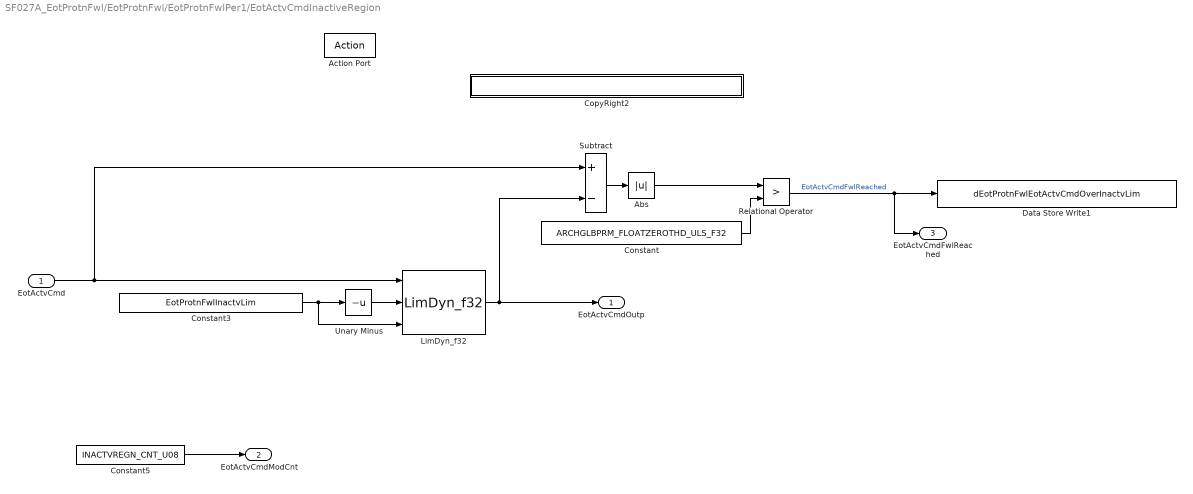
== system SF027A_EotProtnFwl/EotProtnFwl/EotProtnFwlPer1/EotActvCmdInactiveRegion ==
  EotActvCmd : Inport
  Action Port : ActionPort  ActionType=else
  Abs : Abs
  Constant : Constant  Value=ARCHGLBPRM_FLOATZEROTHD_ULS_F32
  Constant3 : Constant  RequirementInfo={} %GIDa_b4942e1c_604a_4bc2_ba0b_2434b0fbe24c  Value=EotProtnFwlInactvLim
  Constant5 : Constant  Value=INACTVREGN_CNT_U08  OutDataTypeStr=uint8
      settings: AttributesFormatString=%<OutDataTypeStr>
  CopyRight2 : Subsystem  Description=|  mask(Copyright Information){none=on}
      | Copyright info block.                                               
      |                                                                     
      | Place copyright information at the top of every subsystem in design.
      mask prompts: none "No parameters"
      mask help: Place copyright information at the top of every subsystem in design.
      mask Display:
      | NxtrConf = 'Nexteer Confidential';
      | 
      | sys = bdroot; %handle for the current model ("system")
      | first = get_param(sys,'Created');
      | first = first(end-3:end);  %year is last four digits
      | 
      | last = get_param(sys,'LastModifiedDate');
      | if isempty(last)
      |     last = datestr(now,'yyyy');
      | else
      |     last = last(end-3:end);
      | end
      | 
      | if strcmp(first,last)
      |     fprintf('%s -- Copyright %s Nexteer',NxtrConf,first)
      | else
      |     fprintf('%s -- %s%s- %s Nexteer',NxtrConf,char(169),first,last)
      | end
  Data Store Write1 : DataStoreWrite  DataStoreName=dEotProtnFwlEotActvCmdOverInactvLim
  LimDyn_f32 : NxtrLim/LimDyn_f32
  Relational Operator : RelationalOperator  Operator=>  OutDataTypeStr=boolean
  Subtract : Sum  Inputs=+-
  Unary Minus : UnaryMinus  RequirementInfo={} %GIDa_9b66f8b9_a3b0_4eb7_9369_8b77fd7e957c
  EotActvCmdOutp : Outport
  EotActvCmdModCnt : Outport  Port=2  InitialOutput=0
  EotActvCmdFwlReached : Outport  Port=3
      settings: AttributesFormatString=%<Tag>
  wires:
  EotActvCmd/1 -> Subtract/1, LimDyn_f32/1
  Relational Operator/1 -> EotActvCmdFwlReached/1, Data Store Write1/1  "EotActvCmdFwlReached"
  Unary Minus/1 -> LimDyn_f32/2
  Constant3/1 -> LimDyn_f32/3, Unary Minus/1
  LimDyn_f32/1 -> Subtract/2, EotActvCmdOutp/1
  Constant5/1 -> EotActvCmdModCnt/1
  Subtract/1 -> Abs/1
  Abs/1 -> Relational Operator/1
  Constant/1 -> Relational Operator/2

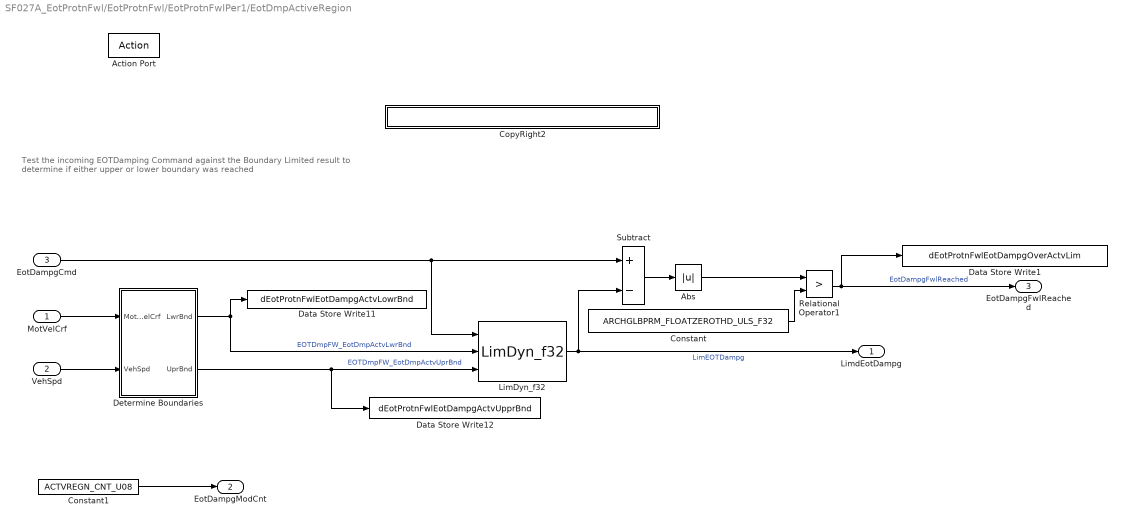
== system SF027A_EotProtnFwl/EotProtnFwl/EotProtnFwlPer1/EotDmpActiveRegion ==
  note: Test the incoming EOTDamping Command against the Boundary Limited result
      | to determine if either upper or lower boundary was reached
  MotVelCrf : Inport
  VehSpd : Inport  Port=2
  EotDampgCmd : Inport  Port=3
  Action Port : ActionPort  ActionType=elseif
  Abs : Abs
  Constant : Constant  Value=ARCHGLBPRM_FLOATZEROTHD_ULS_F32
  Constant1 : Constant  Value=ACTVREGN_CNT_U08  OutDataTypeStr=uint8
      settings: AttributesFormatString=%<OutDataTypeStr>
  CopyRight2 : Subsystem  Description=|  mask(Copyright Information){none=on}
      | Copyright info block.                                               
      |                                                                     
      | Place copyright information at the top of every subsystem in design.
      mask prompts: none "No parameters"
      mask help: Place copyright information at the top of every subsystem in design.
      mask Display:
      | NxtrConf = 'Nexteer Confidential';
      | 
      | sys = bdroot; %handle for the current model ("system")
      | first = get_param(sys,'Created');
      | first = first(end-3:end);  %year is last four digits
      | 
      | last = get_param(sys,'LastModifiedDate');
      | if isempty(last)
      |     last = datestr(now,'yyyy');
      | else
      |     last = last(end-3:end);
      | end
      | 
      | if strcmp(first,last)
      |     fprintf('%s -- Copyright %s Nexteer',NxtrConf,first)
      | else
      |     fprintf('%s -- %s%s- %s Nexteer',NxtrConf,char(169),first,last)
      | end
  Data Store Write1 : DataStoreWrite  DataStoreName=dEotProtnFwlEotDampgOverActvLim
  Data Store Write11 : DataStoreWrite  DataStoreName=dEotProtnFwlEotDampgActvLowrBnd
  Data Store Write12 : DataStoreWrite  DataStoreName=dEotProtnFwlEotDampgActvUpprBnd
  Determine Boundaries : Subsystem
  LimDyn_f32 : NxtrLim/LimDyn_f32
  Relational Operator1 : RelationalOperator  Operator=>  OutDataTypeStr=boolean
  Subtract : Sum  Inputs=+-
  LimdEotDampg : Outport
  EotDampgModCnt : Outport  Port=2  InitialOutput=1
  EotDampgFwlReached : Outport  Port=3
      settings: AttributesFormatString=%<Tag>
  wires:
  MotVelCrf/1 -> Determine Boundaries/1(MotVelCrf)
  Determine Boundaries/1(LwrBnd) -> LimDyn_f32/2, Data Store Write11/1  "EOTDmpFW_EotDmpActvLwrBnd"
  Determine Boundaries/2(UprBnd) -> Data Store Write12/1, LimDyn_f32/3  "EOTDmpFW_EotDmpActvUprBnd"
  VehSpd/1 -> Determine Boundaries/2(VehSpd)
  EotDampgCmd/1 -> Subtract/1, LimDyn_f32/1
  LimDyn_f32/1 -> Subtract/2, LimdEotDampg/1  "LimEOTDampg"
  Relational Operator1/1 -> Data Store Write1/1, EotDampgFwlReached/1  "EotDampgFwlReached"
  Constant1/1 -> EotDampgModCnt/1
  Subtract/1 -> Abs/1
  Abs/1 -> Relational Operator1/1
  Constant/1 -> Relational Operator1/2

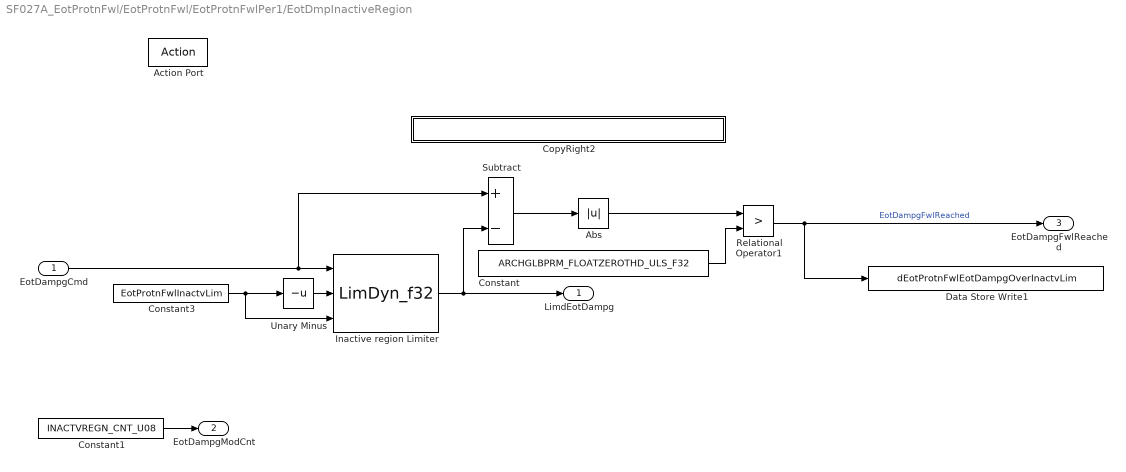
== system SF027A_EotProtnFwl/EotProtnFwl/EotProtnFwlPer1/EotDmpInactiveRegion ==
  EotDampgCmd : Inport
  Action Port : ActionPort  ActionType=else
  Abs : Abs
  Constant : Constant  Value=ARCHGLBPRM_FLOATZEROTHD_ULS_F32
  Constant1 : Constant  Value=INACTVREGN_CNT_U08  OutDataTypeStr=uint8
      settings: AttributesFormatString=%<OutDataTypeStr>
  Constant3 : Constant  RequirementInfo={} %GIDa_51d48208_5135_4d72_ad30_f82a58f3b94c  Value=EotProtnFwlInactvLim
  CopyRight2 : Subsystem  Description=|  mask(Copyright Information){none=on}
      | Copyright info block.                                               
      |                                                                     
      | Place copyright information at the top of every subsystem in design.
      mask prompts: none "No parameters"
      mask help: Place copyright information at the top of every subsystem in design.
      mask Display:
      | NxtrConf = 'Nexteer Confidential';
      | 
      | sys = bdroot; %handle for the current model ("system")
      | first = get_param(sys,'Created');
      | first = first(end-3:end);  %year is last four digits
      | 
      | last = get_param(sys,'LastModifiedDate');
      | if isempty(last)
      |     last = datestr(now,'yyyy');
      | else
      |     last = last(end-3:end);
      | end
      | 
      | if strcmp(first,last)
      |     fprintf('%s -- Copyright %s Nexteer',NxtrConf,first)
      | else
      |     fprintf('%s -- %s%s- %s Nexteer',NxtrConf,char(169),first,last)
      | end
  Data Store Write1 : DataStoreWrite  DataStoreName=dEotProtnFwlEotDampgOverInactvLim
  Inactive region Limiter : NxtrLim/LimDyn_f32
  Relational Operator1 : RelationalOperator  Operator=>  OutDataTypeStr=boolean
  Subtract : Sum  Inputs=+-
  Unary Minus : UnaryMinus  RequirementInfo={} %GIDa_2edc3e87_7cef_48b4_82c5_5f674b7470fc
  LimdEotDampg : Outport
  EotDampgModCnt : Outport  Port=2  InitialOutput=0
  EotDampgFwlReached : Outport  Port=3
      settings: AttributesFormatString=%<Tag>
  wires:
  EotDampgCmd/1 -> Subtract/1, Inactive region Limiter/1
  Relational Operator1/1 -> Data Store Write1/1, EotDampgFwlReached/1  "EotDampgFwlReached"
  Constant1/1 -> EotDampgModCnt/1
  Unary Minus/1 -> Inactive region Limiter/2
  Constant3/1 -> Unary Minus/1, Inactive region Limiter/3
  Inactive region Limiter/1 -> Subtract/2, LimdEotDampg/1
  Subtract/1 -> Abs/1
  Abs/1 -> Relational Operator1/1
  Constant/1 -> Relational Operator1/2
